simulink model "door"  (R2017b)
settings: Solver=VariableStepAuto  StartTime=0.0  StopTime=10  RelTol=1e-3  EnableMultiTasking=on
libraries: simulink x1
settings Model: Creator=user  LastModifiedBy=jessl
settings DataIOCC: LimitDataPoints=on
settings OptimizationCC: LifeSpan=inf
settings DebuggingCC: AllowSymbolicDim=off  SFUnexpectedBacktrackingDiag=warning  SFNoUnconditionalDefaultTransitionDiag=warning  SFExecutionAtInitializationDiag=none
settings ModelReferenceCC: PropagateSignalLabelsOutOfModel=off
settings CodeAppCC: StateflowObjectComments=on
settings GRTTargetCC: TargetLangStandard=C89/C90 (ANSI)
settings ConfigComp: CovMetricSettings=dw  CovHtmlReporting=on  CovSaveCumulativeToWorkspaceVar=on  CovSaveSingleToWorkspaceVar=on  CovExternalEMLEnable=off

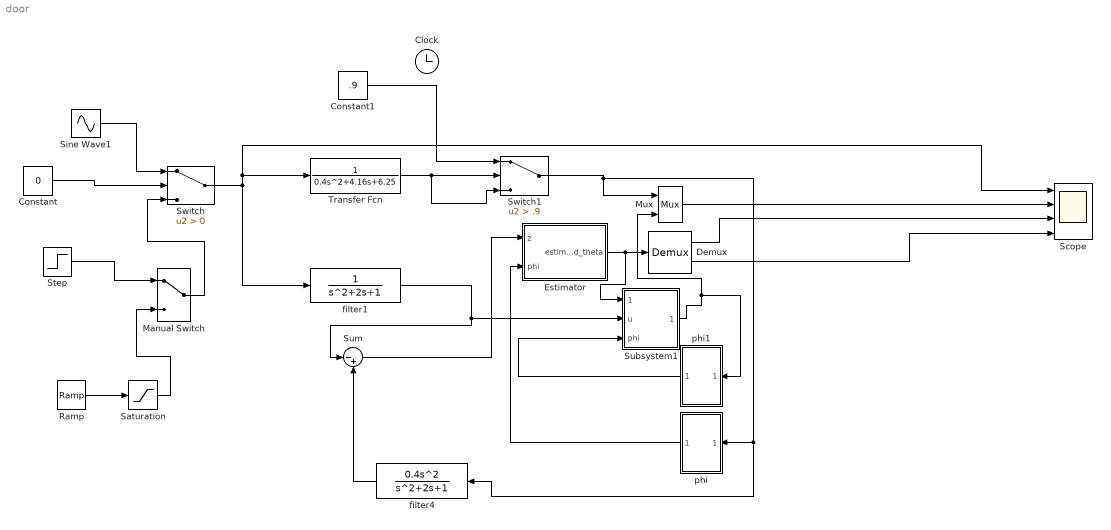
== system door ==
  Clock : Clock
      settings: Decimation=250
  Constant : Constant  Value=0
  Constant1 : Constant  Value=.9
  Demux : Demux  Outputs=2
  Estimator : Subsystem
      mask Display: disp('Parameter\nEstimation')
  Manual Switch : ManualSwitch
  Mux : Mux  Inputs=2
  Ramp : simulink/Sources/Ramp  slope=1  start=0  X0=0
  Saturation : Saturate  UpperLimit=9.81/1.5
  Scope : Scope  NumInputPorts=4
  Sine Wave1 : Sin  Bias=1  Frequency=pi/3  Phase=pi/2  SampleTime=0
  Step : Step  After=9.81/1.5  SampleTime=0.001
  Subsystem1 : Subsystem
  Sum : Sum  Inputs=|-+
  Switch : Switch  Criteria=u2 > Threshold
  Switch1 : Switch  Criteria=u2 > Threshold  Threshold=.9
  Transfer Fcn : TransferFcn  Denominator=[0.4 4.16 6.25]
  filter1 : TransferFcn
  filter4 : TransferFcn  Numerator=[0.4 0 0]
  phi : Subsystem
  phi1 : Subsystem
  wires:
  phi/1(Out1) -> Estimator/2(phi)
  Transfer Fcn/1 -> Switch1/3, Switch1/2
  filter4/1 -> Sum/2
  filter1/1 -> Sum/1, Subsystem1/2(u)
  Sum/1 -> Estimator/1(z)
  Estimator/1(estimated_theta) -> Subsystem1/1(theta_hat), Demux/1
  Demux/1 -> Scope/3
  Demux/2 -> Scope/4
  Mux/1 -> Scope/2
  Subsystem1/1(x_hat) -> phi1/1(In1), Mux/2
  phi1/1(Out1) -> Subsystem1/3(phi)
  Switch/1 -> Transfer Fcn/1, Scope/1, filter1/1
  Sine Wave1/1 -> Switch/1
  Constant/1 -> Switch/2
  Ramp/1 -> Saturation/1
  Step/1 -> Manual Switch/1
  Saturation/1 -> Manual Switch/2
  Manual Switch/1 -> Switch/3
  Switch1/1 -> filter4/1, phi/1(In1), Mux/1
  Constant1/1 -> Switch1/1

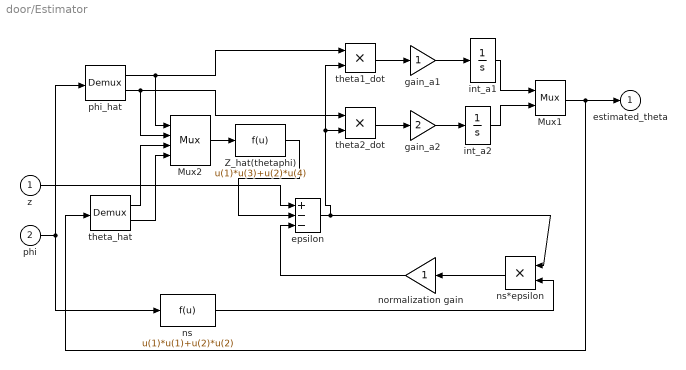
== system door/Estimator ==
  z : Inport
  phi : Inport  Port=2
  Mux1 : Mux  Inputs=2
  Mux2 : Mux
  Z_hat(thetaphi) : Fcn  Expr=u(1)*u(3)+u(2)*u(4)
  epsilon : Sum  Inputs=+--  SaturateOnIntegerOverflow=on  InputSameDT=on  OutDataTypeStr=Inherit: Same as first input
  gain_a1 : Gain  SaturateOnIntegerOverflow=on  OutDataTypeStr=Inherit: Same as input  ParamDataTypeStr=Inherit: Same as input
  gain_a2 : Gain  Gain=2  SaturateOnIntegerOverflow=on  OutDataTypeStr=Inherit: Same as input  ParamDataTypeStr=Inherit: Same as input
  int_a1 : Integrator
  int_a2 : Integrator
  normalization gain : Gain  SaturateOnIntegerOverflow=on  OutDataTypeStr=Inherit: Same as input  ParamDataTypeStr=Inherit: Same as input
  ns : Fcn  Expr=u(1)*u(1)+u(2)*u(2)
      mask Display: disp('phi ''phi')
  ns*epsilon : Product  SaturateOnIntegerOverflow=on  RndMeth=Zero  InputSameDT=on  OutDataTypeStr=Inherit: Same as first input
  phi_hat : Demux  Outputs=2
  theta1_dot : Product  SaturateOnIntegerOverflow=on  RndMeth=Zero  InputSameDT=on  OutDataTypeStr=Inherit: Same as first input
  theta2_dot : Product  SaturateOnIntegerOverflow=on  RndMeth=Zero  InputSameDT=on  OutDataTypeStr=Inherit: Same as first input
  theta_hat : Demux  Outputs=2
  estimated_theta : Outport
  wires:
  z/1 -> epsilon/1
  normalization gain/1 -> epsilon/3
  phi_hat/1 -> theta1_dot/1, Mux2/1
  phi_hat/2 -> theta2_dot/1, Mux2/2
  Mux1/1 -> estimated_theta/1, theta_hat/1
  Z_hat(thetaphi)/1 -> epsilon/2
  phi/1 -> ns/1, phi_hat/1
  epsilon/1 -> ns*epsilon/1, theta1_dot/2, theta2_dot/2
  ns*epsilon/1 -> normalization gain/1
  int_a1/1 -> Mux1/1
  int_a2/1 -> Mux1/2
  theta_hat/1 -> Mux2/3
  theta_hat/2 -> Mux2/4
  Mux2/1 -> Z_hat(thetaphi)/1
  theta2_dot/1 -> gain_a2/1
  gain_a2/1 -> int_a2/1
  theta1_dot/1 -> gain_a1/1
  gain_a1/1 -> int_a1/1
  ns/1 -> ns*epsilon/2

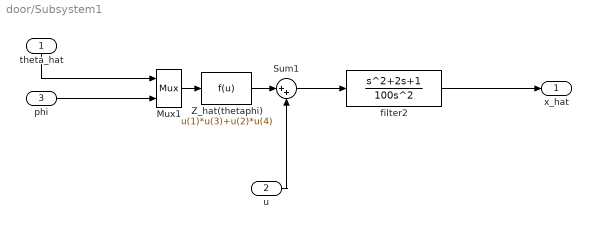
== system door/Subsystem1 ==
  theta_hat : Inport
  u : Inport  Port=2
  phi : Inport  Port=3
  Mux1 : Mux  Inputs=2
  Sum1 : Sum  Inputs=|++
  Z_hat(thetaphi) : Fcn  Expr=u(1)*u(3)+u(2)*u(4)
  filter2 : TransferFcn  Numerator=[1 2 1]  Denominator=[100 0 0]
  x_hat : Outport
  wires:
  phi/1 -> Mux1/2
  u/1 -> Sum1/2
  theta_hat/1 -> Mux1/1
  filter2/1 -> x_hat/1
  Mux1/1 -> Z_hat(thetaphi)/1
  Sum1/1 -> filter2/1
  Z_hat(thetaphi)/1 -> Sum1/1

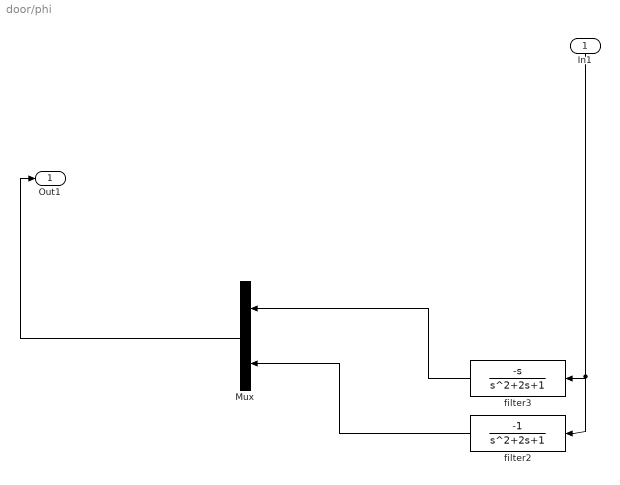
== system door/phi ==
  In1 : Inport
  Mux : Mux  Inputs=2
  filter2 : TransferFcn  Numerator=[-1 ]
  filter3 : TransferFcn  Numerator="[-1  0]"
  Out1 : Outport
  wires:
  In1/1 -> filter2/1, filter3/1
  filter2/1 -> Mux/2
  Mux/1 -> Out1/1
  filter3/1 -> Mux/1

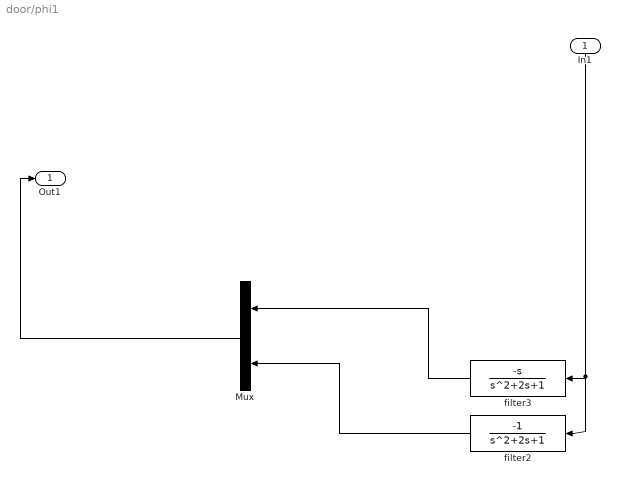
== system door/phi1 ==
  In1 : Inport
  Mux : Mux  Inputs=2
  filter2 : TransferFcn  Numerator=[-1 ]
  filter3 : TransferFcn  Numerator="[-1  0]"
  Out1 : Outport
  wires:
  In1/1 -> filter2/1, filter3/1
  filter2/1 -> Mux/2
  Mux/1 -> Out1/1
  filter3/1 -> Mux/1
